simulink model "object_tracker_intensity"  (Simulink 6.4)
settings: Solver=FixedStepDiscrete  StartTime=0.0  StopTime=inf  RelTol=1e-3
StartFcn:
  | ppo_start
StopFcn:
  | ppo_stop
model workspace: external: M-Code (data not in the file)
undefined symbols (not defined in the file or in its folder): Kanade, line_row, Lucas, Rec, SDTV
libraries: viptextngfix x9, dspmtrx3 x7, vipsnks x5, vipconversions x3, vipanalysis x2, simulink x2, vipstatistics x1, vipmisc x1, dspindex x1, imaqlib x1
settings Model: Creator=don  LastModifiedBy=Raza  ExtModeAutoUpdateStatusClock=off
settings DataIOCC: LimitDataPoints=off  SaveOutput=off  SignalLogging=off  SaveTime=off  SignalLoggingName=sigsOut
settings OptimizationCC: BufferReusableBoundary=off
settings DebuggingCC: AlgebraicLoopMsg=none  CheckExecutionContextPreStartOutputMsg=on  CheckExecutionContextRuntimeOutputMsg=on  SolverPrmCheckMsg=none  SigSpecEnsureSampleTimeMsg=none  ParameterPrecisionLossMsg=none  BusObjectLabelMismatch=none  StrictBusMsg=None
settings HardwareCC: TargetHWDeviceType=32-bit Generic  ProdEqTarget=off

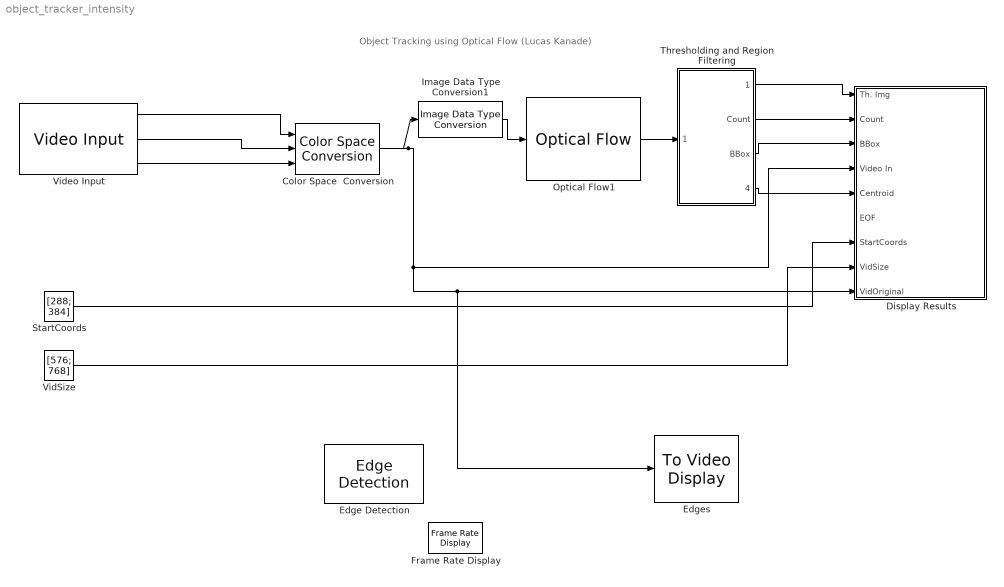
== system object_tracker_intensity ==
  note: Object Tracking using Optical Flow (Lucas Kanade)
  Color Space  Conversion : vipconversions/Color Space  Conversion  conversion=R'G'B' to intensity  wp_str=D65  rec=Rec. 601 (SDTV)  sys=1125/60/2:1
  Display Results : Subsystem
  Edge Detection : vipanalysis/Edge Detection  DialogController=vipDDGCreate  DialogControllerArgs=DataTag2  method=Prewitt  outputType=Binary image  userDefinedThreshold=on  thresholdSource=Specify via dialog  threshold=0.06  thresholdTuning=10  edgeThinning=on  threshold_canny=[0.25 0.60]  autoPercent=70  sigma=3  roundingMode=Floor  overflowMode=off
  Edges : vipsnks/To Video Display  inputType=Intensity  OutputDevice=On-screen video monitor  fullScreen=off  videoWindowX=89  videoWindowY=69  saveWindowSize=off  videoWindowWidth=776  videoWindowHeight=603
  Frame Rate Display : vipsnks/Frame Rate Display  DialogController=vipDDGCreate  DialogControllerArgs=DataTag3  UpdateRate=10
  Image Data Type Conversion1 : vipconversions/Image Data Type Conversion  outDT=double  isSigned=on  wordLen=16  numFracBits=0
  Optical Flow1 : vipanalysis/Optical Flow  SystemSampleTime=-1  method=Lucas-Kanade  which2img=Current frame and N-th frame back  N=1  outVelForm=Magnitude-squared  lambda=1  stop_criteria=When maximum number of iterations is reached  maxAllowAbsDiff=eps  maxIter=10  eigTh=0.007
  StartCoords : Constant  Value=[288; 384]  OutDataTypeMode=uint16  OutDataType=sfix(16)  ConRadixGroup=Use specified scaling  OutScaling=2^0  SampleTime=inf  FramePeriod=inf
      settings: SamplingMode=Frame based
  Thresholding and Region Filtering : Subsystem
  VidSize : Constant  Value=[576; 768]  OutDataTypeMode=uint16  OutDataType=sfix(16)  ConRadixGroup=Use specified scaling  OutScaling=2^0  SampleTime=inf  FramePeriod=inf
      settings: SamplingMode=Frame based
  Video Input : imaqlib/Video Input  DialogController=imaqcreatedialog  DialogControllerArgs=DataTag5  VideoDeviceMenu=1 (Bt878 TV Card)  VideoDevice=1 (Bt878 TV Card)  VideoStreamFormatMenu=RGB555_768x576  VideoStreamFormat=RGB555_768x576  VideoFrameSizeMenu=INPUTSIZE  VideoFrameSize=INPUTSIZE  FrameRate=30 fps  DataType=uint8
  wires:
  Thresholding and Region Filtering/3(BBox) -> Display Results/3(BBox)
  Thresholding and Region Filtering/2(Count) -> Display Results/2(Count)
  Thresholding and Region Filtering/4(Centroid) -> Display Results/5(Centroid)
  StartCoords/1 -> Display Results/7(StartCoords)
  VidSize/1 -> Display Results/8(VidSize)
  Optical Flow1/1 -> Thresholding and Region Filtering/1(Sq. Mag)
  Color Space  Conversion/1 -> Display Results/4(Video In), Display Results/9(VidOriginal), Edges/1, Image Data Type Conversion1/1
  Thresholding and Region Filtering/1(Th. Img) -> Display Results/1(Th. Img)
  Video Input/2 -> Color Space  Conversion/2
  Video Input/3 -> Color Space  Conversion/3
  Video Input/1 -> Color Space  Conversion/1
  Image Data Type Conversion1/1 -> Optical Flow1/1

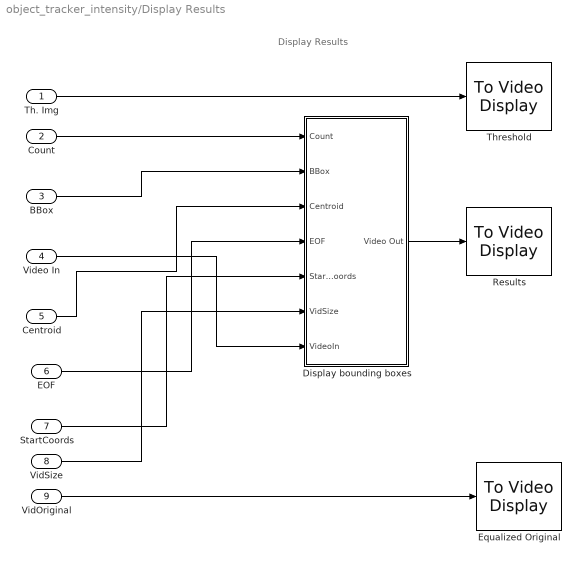
== system object_tracker_intensity/Display Results ==
  note: Display Results
  Th. Img : Inport
  Count : Inport  Port=2
  BBox : Inport  Port=3
  Video In : Inport  Port=4
  Centroid : Inport  Port=5
  EOF : Inport  Port=6
  StartCoords : Inport  Port=7
  VidSize : Inport  Port=8
  VidOriginal : Inport  Port=9
  Display bounding boxes : Subsystem
  Equalized Original : vipsnks/To Video Display  inputType=Intensity  OutputDevice=On-screen video monitor  fullScreen=off  videoWindowX=200  videoWindowY=33  saveWindowSize=off  videoWindowWidth=776  videoWindowHeight=603
  Results : vipsnks/To Video Display  inputType=Intensity  OutputDevice=On-screen video monitor  fullScreen=off  videoWindowX=404  videoWindowY=129  saveWindowSize=off  videoWindowWidth=776  videoWindowHeight=603
  Threshold : vipsnks/To Video Display  inputType=Intensity  OutputDevice=On-screen video monitor  fullScreen=off  videoWindowX=464  videoWindowY=37  saveWindowSize=off  videoWindowWidth=776  videoWindowHeight=603
  wires:
  Th. Img/1 -> Threshold/1
  Count/1 -> Display bounding boxes/1(Count)
  BBox/1 -> Display bounding boxes/2(BBox)
  Centroid/1 -> Display bounding boxes/3(Centroid)
  Display bounding boxes/1(Video Out) -> Results/1
  EOF/1 -> Display bounding boxes/4(EOF)
  StartCoords/1 -> Display bounding boxes/5(StartCoords)
  VidSize/1 -> Display bounding boxes/6(VidSize)
  VidOriginal/1 -> Equalized Original/1
  Video In/1 -> Display bounding boxes/7(VideoIn)

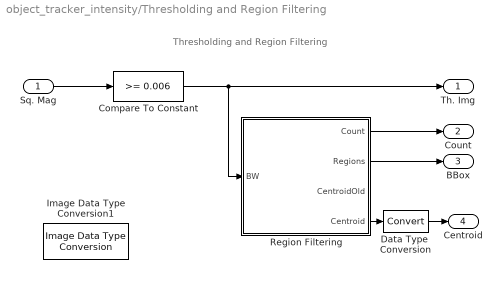
== system object_tracker_intensity/Thresholding and Region Filtering ==
  note: Thresholding and Region Filtering
  Sq. Mag : Inport
  Compare To Constant : simulink/Logic and Bit Operations/Compare To Constant  SystemSampleTime=-1  relop=>=  const=0.006  LogicOutDataTypeMode=boolean
  Data Type  Conversion : DataTypeConversion  OutDataTypeMode=uint16  SaturateOnIntegerOverflow=on  RndMeth=Zero
  Image Data Type Conversion1 : vipconversions/Image Data Type Conversion  outDT=uint16  isSigned=on  wordLen=16  numFracBits=0
  Region Filtering : Subsystem
  Th. Img : Outport
  Count : Outport  Port=2
  BBox : Outport  Port=3
  Centroid : Outport  Port=4
  wires:
  Compare To Constant/1 -> Region Filtering/1(BW), Th. Img/1
  Sq. Mag/1 -> Compare To Constant/1
  Region Filtering/1(Count) -> Count/1
  Region Filtering/2(Regions) -> BBox/1
  Region Filtering/4(Centroid) -> Data Type  Conversion/1
  Data Type  Conversion/1 -> Centroid/1

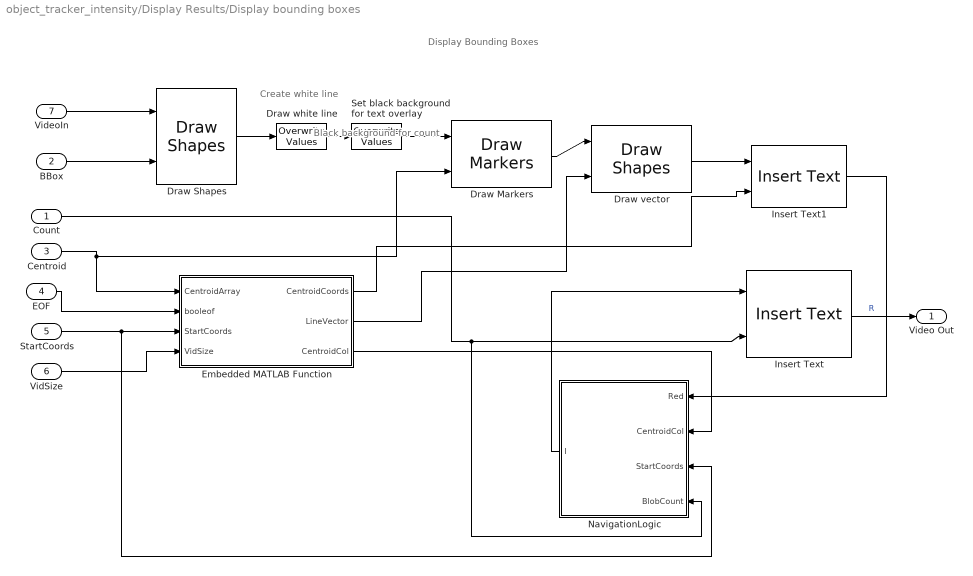
== system object_tracker_intensity/Display Results/Display bounding boxes ==
  note: Black background
      | for count
  note: Create white
      | line
  note: Display Bounding Boxes
  Count : Inport
  BBox : Inport  Port=2
  Centroid : Inport  Port=3
  EOF : Inport  Port=4
  StartCoords : Inport  Port=5
  VidSize : Inport  Port=6
  VideoIn : Inport  Port=7
  Draw Markers : viptextngfix/Draw Markers  inType=Intensity  shape=X-mark  size=3  fill=off  display=White  intensity=155  color=[200 120 50]  opacity=1  viewport=Entire image
  Draw Shapes : viptextngfix/Draw Shapes  DialogController=vipDDGCreate  DialogControllerArgs=DataTag0  inType=Intensity  shape=Rectangles  fill=off  display=User-specified value  intensity=200  color=[0 1 0]  opacity=0.6  viewport=Entire image  antialiasing=off
  Draw vector : viptextngfix/Draw Shapes  DialogController=vipDDGCreate  DialogControllerArgs=DataTag1  inType=Intensity  shape=Lines  fill=off  display=White  intensity=200  color=[200 255 100]  opacity=0.6  viewport=Entire image  antialiasing=off
  Draw white line : dspmtrx3/Overwrite Values  OverWriteDiag=Submatrix  valFrom2ndIP=Specify via dialog  ConstValue=1  RowSpan=Range of rows  RowStartMode=Index  RowStartIndex=22  RowEndMode=Index  RowEndIndex=22+1  ColSpan=All columns  ColStartMode=First  ColStartIndex=1  ColEndMode=Last  ColEndIndex=1  DiagSpan=Range of elements  DiagStartMode=Index  DiagStartIndex=2  DiagEndMode=Index  DiagEndIndex=4
  Embedded MATLAB Function : Stateflow chart
  Insert Text : viptextngfix/Insert Text  inputType=Intensity  theText='%4d'  fontFace=Arial  dummyVar1=0  blockFontSize=12  antiAliased=on  getTextLocFrom=Specify via dialog  textLoc=[0 0]  getTextColorFrom=Specify via dialog  textColor=[1 1 1]  getTextIntensityFrom=Specify via dialog  textIntensity=1  getTextOpacityFrom=Specify via dialog  textOpacity=1.0  dummyVar2=0  dummyVar3=0  dummyVar4=0
  Insert Text1 : viptextngfix/Insert Text  inputType=Intensity  theText='(%2.0f,%2.0f)'  fontFace=Arial  dummyVar1=0  blockFontSize=12  antiAliased=on  getTextLocFrom=Specify via dialog  textLoc=[0 40]  getTextColorFrom=Specify via dialog  textColor=[1 1 1]  getTextIntensityFrom=Specify via dialog  textIntensity=1  getTextOpacityFrom=Specify via dialog  textOpacity=1.0  dummyVar2=0  dummyVar3=0  dummyVar4=0
  NavigationLogic : Subsystem  Orientation=left
  Set black background for text overlay : dspmtrx3/Overwrite Values  OverWriteDiag=Submatrix  valFrom2ndIP=Specify via dialog  ConstValue=0  RowSpan=Range of rows  RowStartMode=First  RowStartIndex=25  RowEndMode=Index  RowEndIndex=15  ColSpan=Range of columns  ColStartMode=First  ColStartIndex=1  ColEndMode=Index  ColEndIndex=30  DiagSpan=Range of elements  DiagStartMode=Index  DiagStartIndex=2  DiagEndMode=Index  DiagEndIndex=4
  Video Out : Outport
  wires:
  Draw white line/1 -> Set black background for text overlay/1
  Centroid/1 -> Embedded MATLAB Function/1(CentroidArray), Draw Markers/2
  Set black background for text overlay/1 -> Draw Markers/1
  Draw Markers/1 -> Draw vector/1
  Draw vector/1 -> Insert Text1/1
  Insert Text1/1 -> NavigationLogic/1(Red)
  EOF/1 -> Embedded MATLAB Function/2(booleof)
  StartCoords/1 -> Embedded MATLAB Function/3(StartCoords), NavigationLogic/3(StartCoords)
  VidSize/1 -> Embedded MATLAB Function/4(VidSize)
  Embedded MATLAB Function/3(CentroidCol) -> NavigationLogic/2(CentroidCol)
  Embedded MATLAB Function/1(CentroidCoords) -> Insert Text1/2
  Count/1 -> NavigationLogic/4(BlobCount), Insert Text/2
  NavigationLogic/1(I) -> Insert Text/1
  VideoIn/1 -> Draw Shapes/1
  BBox/1 -> Draw Shapes/2
  Draw Shapes/1 -> Draw white line/1
  Embedded MATLAB Function/2(LineVector) -> Draw vector/2
  Insert Text/1 -> Video Out/1  "R"

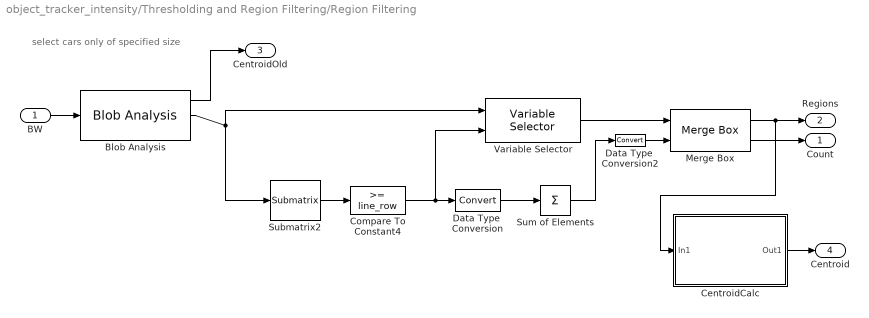
== system object_tracker_intensity/Thresholding and Region Filtering/Region Filtering ==
  note: select cars only of specified size
  BW : Inport
  Blob Analysis : vipstatistics/Blob Analysis  DialogController=vipDDGCreate  DialogControllerArgs=DataTag4  area=off  centroid=on  bBox=on  majorAxis=off  minorAxis=off  angle=off  eccentricity=off  equivDiameterSq=off  extent=off  perimeter=off  maxBlobs=10  warnIfNumBlobsExceeded=on  isCount=on  useMinArea=on  minArea=100  useMaxArea=on  maxArea=2500  excludeBorderBlob=off  outDT=double  isFill=on  fillValues=-1  conn=8  isLabel=off  outputMode=Binary point scaling  outputWordLength=32  outputFracLength=16  firstCoeffMode=Binary point scaling  firstCoeffWordLength=16  firstCoeffFracLength=14  secondCoeffMode=Binary point scaling  secondCoeffWordLength=32  secondCoeffFracLength=16  accumMode=Binary point scaling  accumWordLength=32  accumFracLength=0  prodOutputMode=Binary point scaling  prodOutputWordLength=32  prodOutputFracLength=16  roundingMode=Floor  overflowMode=off
  CentroidCalc : Subsystem
  Compare To Constant4 : simulink/Logic and Bit Operations/Compare To Constant  SystemSampleTime=-1  relop=>=  const=line_row  LogicOutDataTypeMode=boolean  ZeroCross=off
  Data Type  Conversion : DataTypeConversion  OutDataTypeMode=single  SaturateOnIntegerOverflow=on  RndMeth=Zero
  Data Type  Conversion2 : DataTypeConversion  OutDataTypeMode=int32  SaturateOnIntegerOverflow=on  RndMeth=Zero
  Merge Box : vipmisc/Merge Box  whichdir=Row direction only  cdist=60  rdist=45
  Submatrix2 : dspmtrx3/Submatrix  RowSpan=One row  RowStartMode=Index  RowStartIndex=1  RowEndMode=Last  RowEndIndex=1  ColSpan=All columns  ColStartMode=First  ColStartIndex=1  ColEndMode=Last  ColEndIndex=1
  Sum of Elements : Sum  Inputs=+  OutScaling=2^-10
  Variable Selector : dspindex/Variable Selector  NumInputs=1  rowsOrCols=Columns  IdxMode=Variable  Elements=[1 3]  ZerOneIdxMode=Zero-based  errmode=Clip Index  FillMode=on  FillValues=-1
  Count : Outport
  Regions : Outport  Port=2
  CentroidOld : Outport  Port=3
  Centroid : Outport  Port=4
  wires:
  Data Type  Conversion/1 -> Sum of Elements/1
  Sum of Elements/1 -> Data Type  Conversion2/1
  Compare To Constant4/1 -> Data Type  Conversion/1, Variable Selector/2
  Submatrix2/1 -> Compare To Constant4/1
  BW/1 -> Blob Analysis/1
  Variable Selector/1 -> Merge Box/1
  Merge Box/1 -> Regions/1, CentroidCalc/1(In1)
  Merge Box/2 -> Count/1
  Data Type  Conversion2/1 -> Merge Box/2
  Blob Analysis/2 -> Submatrix2/1, Variable Selector/1
  Blob Analysis/1 -> CentroidOld/1
  CentroidCalc/1(Out1) -> Centroid/1

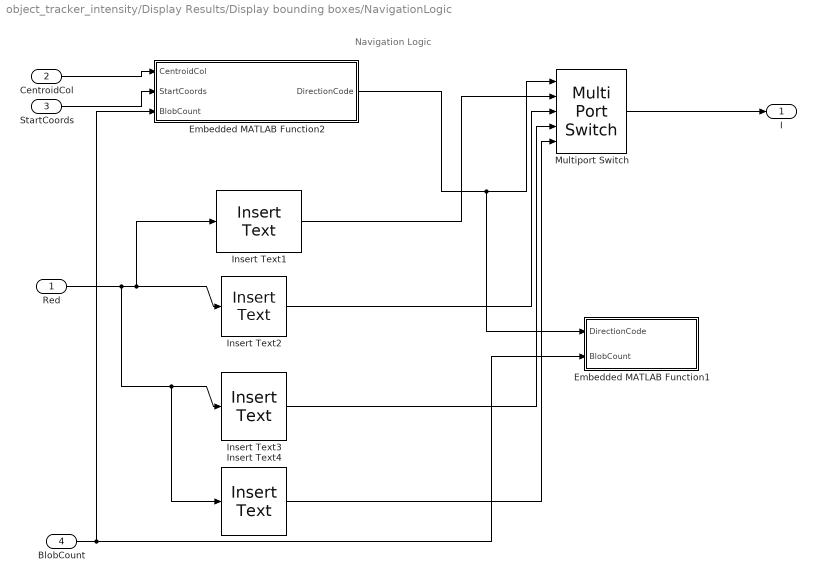
== system object_tracker_intensity/Display Results/Display bounding boxes/NavigationLogic ==
  note: Navigation Logic
  Red : Inport
  CentroidCol : Inport  Port=2
  StartCoords : Inport  Port=3
  BlobCount : Inport  Port=4
  Embedded MATLAB Function1 : Stateflow chart
  Embedded MATLAB Function2 : Stateflow chart
  Insert Text1 : viptextngfix/Insert Text  inputType=Intensity  theText='STRAIGHT'  fontFace=Arial  dummyVar1=0  blockFontSize=12  antiAliased=on  getTextLocFrom=Specify via dialog  textLoc=[0 100]  getTextColorFrom=Specify via dialog  textColor=[1 1 1]  getTextIntensityFrom=Specify via dialog  textIntensity=1  getTextOpacityFrom=Specify via dialog  textOpacity=1.0  dummyVar2=0  dummyVar3=0  dummyVar4=0
  Insert Text2 : viptextngfix/Insert Text  inputType=Intensity  theText='LEFT'  fontFace=Arial  dummyVar1=0  blockFontSize=12  antiAliased=on  getTextLocFrom=Specify via dialog  textLoc=[0 100]  getTextColorFrom=Specify via dialog  textColor=[1 1 1]  getTextIntensityFrom=Specify via dialog  textIntensity=1  getTextOpacityFrom=Specify via dialog  textOpacity=1.0  dummyVar2=0  dummyVar3=0  dummyVar4=0
  Insert Text3 : viptextngfix/Insert Text  inputType=Intensity  theText='RIGHT'  fontFace=Arial  dummyVar1=0  blockFontSize=12  antiAliased=on  getTextLocFrom=Specify via dialog  textLoc=[0 100]  getTextColorFrom=Specify via dialog  textColor=[1 1 1]  getTextIntensityFrom=Specify via dialog  textIntensity=1  getTextOpacityFrom=Specify via dialog  textOpacity=1.0  dummyVar2=0  dummyVar3=0  dummyVar4=0
  Insert Text4 : viptextngfix/Insert Text  inputType=Intensity  theText='STOP'  fontFace=Arial  dummyVar1=0  blockFontSize=12  antiAliased=on  getTextLocFrom=Specify via dialog  textLoc=[0 100]  getTextColorFrom=Specify via dialog  textColor=[1 1 1]  getTextIntensityFrom=Specify via dialog  textIntensity=1  getTextOpacityFrom=Specify via dialog  textOpacity=1.0  dummyVar2=0  dummyVar3=0  dummyVar4=0
  Multiport Switch : MultiPortSwitch
  I : Outport
  wires:
  Red/1 -> Insert Text2/1, Insert Text1/1, Insert Text3/1, Insert Text4/1
  Multiport Switch/1 -> I/1
  CentroidCol/1 -> Embedded MATLAB Function2/1(CentroidCol)
  StartCoords/1 -> Embedded MATLAB Function2/2(StartCoords)
  Embedded MATLAB Function2/1(DirectionCode) -> Multiport Switch/1, Embedded MATLAB Function1/1(DirectionCode)
  BlobCount/1 -> Embedded MATLAB Function1/2(BlobCount), Embedded MATLAB Function2/3(BlobCount)
  Insert Text1/1 -> Multiport Switch/2
  Insert Text2/1 -> Multiport Switch/3
  Insert Text3/1 -> Multiport Switch/4
  Insert Text4/1 -> Multiport Switch/5

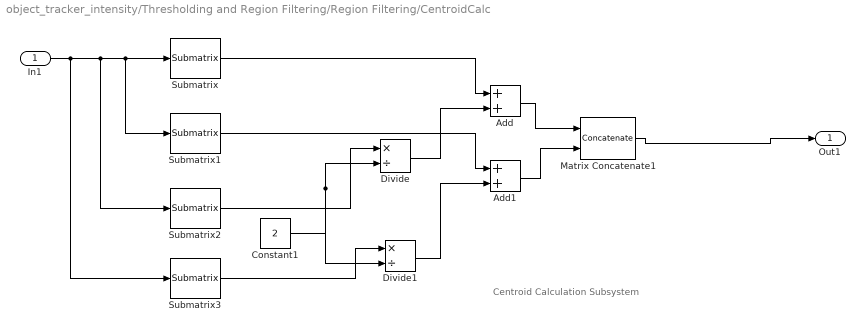
== system object_tracker_intensity/Thresholding and Region Filtering/Region Filtering/CentroidCalc ==
  note: Centroid Calculation
      | Subsystem
  In1 : Inport
  Add : Sum  OutScaling=2^-10
  Add1 : Sum  OutScaling=2^-10
  Constant1 : Constant  Value=2  OutDataType=sfix(16)  ConRadixGroup=Use specified scaling  OutScaling=2^0  SampleTime=inf  FramePeriod=inf
  Divide : Product  Inputs=*/  OutScaling=2^-10
  Divide1 : Product  Inputs=*/  OutScaling=2^-10
  Matrix Concatenate1 : Concatenate  Mode=Vertical matrix concatenation
  Submatrix : dspmtrx3/Submatrix  RowSpan=One row  RowStartMode=Index  RowStartIndex=1  RowEndMode=Last  RowEndIndex=1  ColSpan=All columns  ColStartMode=Offset from last  ColStartIndex=1  ColEndMode=Last  ColEndIndex=1
  Submatrix1 : dspmtrx3/Submatrix  RowSpan=One row  RowStartMode=Index  RowStartIndex=2  RowEndMode=Last  RowEndIndex=1  ColSpan=All columns  ColStartMode=Offset from last  ColStartIndex=1  ColEndMode=Last  ColEndIndex=1
  Submatrix2 : dspmtrx3/Submatrix  RowSpan=One row  RowStartMode=Index  RowStartIndex=3  RowEndMode=Last  RowEndIndex=1  ColSpan=All columns  ColStartMode=Offset from last  ColStartIndex=1  ColEndMode=Last  ColEndIndex=1
  Submatrix3 : dspmtrx3/Submatrix  RowSpan=One row  RowStartMode=Index  RowStartIndex=4  RowEndMode=Last  RowEndIndex=1  ColSpan=All columns  ColStartMode=Offset from last  ColStartIndex=1  ColEndMode=Last  ColEndIndex=1
  Out1 : Outport
  wires:
  Add1/1 -> Matrix Concatenate1/2
  Add/1 -> Matrix Concatenate1/1
  Divide1/1 -> Add1/2
  Submatrix1/1 -> Add1/1
  Divide/1 -> Add/2
  Submatrix/1 -> Add/1
  Submatrix3/1 -> Divide1/1
  Submatrix2/1 -> Divide/1
  Constant1/1 -> Divide/2, Divide1/2
  In1/1 -> Submatrix/1, Submatrix1/1, Submatrix2/1, Submatrix3/1
  Matrix Concatenate1/1 -> Out1/1

== matlab function Display Results/Display bounding boxes/NavigationLogic/Embedded MATLAB Function1 ==
  data: DirectionCode input inherited; BlobCount input inherited
function Turnit(DirectionCode, BlobCount)
% This block supports an embeddable subset of the MATLAB language.
% See the help menu for details. 
DIFFTHING = 5;
BRAKEDIFF = 2;

persistent movecount; %no of frames after which the position of the car is updated.
persistent brakecount;

persistent startflag;

if isempty ( startflag ) 
    startflag = 1;
else
    startflag = 0;
end

if isempty ( brakecount ) 
    brakecount = 0;
end

if  isempty ( movecount ) 
    movecount = 0;
end

if BlobCount == 0 
    movecount = DIFFTHING;
    brakecount = 0;
    startflag = 1;
    BrakeAll;
    return;
end

movecount = movecount + 1;
brakecount = brakecount + 1;

if ( brakecount >= BRAKEDIFF )
    BrakeAll;
end

    
if ( movecount >= DIFFTHING || startflag == 1 )
    
    if  DirectionCode == 1    %Forward
        MoveForward(1);
    elseif  DirectionCode == 2  %Left
        MoveLeft ( 1 );
    elseif DirectionCode == 3  %Right
        MoveRight ( 1 );
    end

    MoveForward(1);
    movecount = 0;

end

== matlab function Display Results/Display bounding boxes/Embedded MATLAB Function ==
  data: CentroidCoords output inherited; CentroidArray input inherited; LineVector output inherited; booleof input inherited; StartCoords input inherited; VidSize input inherited; CentroidCol output inherited
function [CentroidCoords,LineVector, CentroidCol] = ObjectTracker(CentroidArray,booleof,StartCoords,VidSize)
% This block supports an embeddable subset of the MATLAB language.
% See the help menu for details. 
persistent LastCentroid;

if isempty(LastCentroid) || booleof == true
    LastCentroid = StartCoords;
end

z = LastCentroid;

allx = CentroidArray(1,:) - z(1);
ally = CentroidArray(2,:) - z(2);
myvector =  allx.^2 + ally.^2;
[m i] = min (myvector);
centroid = CentroidArray(:,i(1));

if myvector(i(1)) < 10000 && centroid(1) > 0 && centroid(2) > 10
    LastCentroid = centroid;
    CentroidCoords = centroid;
else
    CentroidCoords = z;
end

LineVector = [ VidSize(1) , VidSize(2)/2 , CentroidCoords(1) , CentroidCoords(2) ];
CentroidCol = CentroidCoords(2);

== matlab function Display Results/Display bounding boxes/NavigationLogic/Embedded MATLAB Function2 ==
  data: CentroidCol input inherited; StartCoords input inherited; DirectionCode output inherited; BlobCount input inherited
function DirectionCode = DirectionTest(CentroidCol, StartCoords, BlobCount)

STRAIGHT = 1;
LEFT = 2;
RIGHT = 3;
STOP = 4;

DIFFTHRESHOLD = 20;
ScreenCenter = StartCoords(2);

if BlobCount == 0
    DirectionCode = STOP;
elseif CentroidCol < ScreenCenter - DIFFTHRESHOLD
    DirectionCode = LEFT;
elseif CentroidCol > ScreenCenter + DIFFTHRESHOLD
    DirectionCode = RIGHT;
else
    DirectionCode = STRAIGHT;
end
